simulink model "SimQLPVOFb"  (R2017a)
settings: Solver=VariableStepAuto  StartTime=0.0  StopTime=2000  FixedStep=1e-3  RelTol=1e-3  EnableMultiTasking=on
undefined symbols (not defined in the file): Dr, Du, K, toMpS, toRad, toRPS
libraries: dspsigattribs x3
settings Model: Creator=c00rts11  LastModifiedBy=c00rts11
settings SolverCC: ZeroCrossAlgorithm=Adaptive

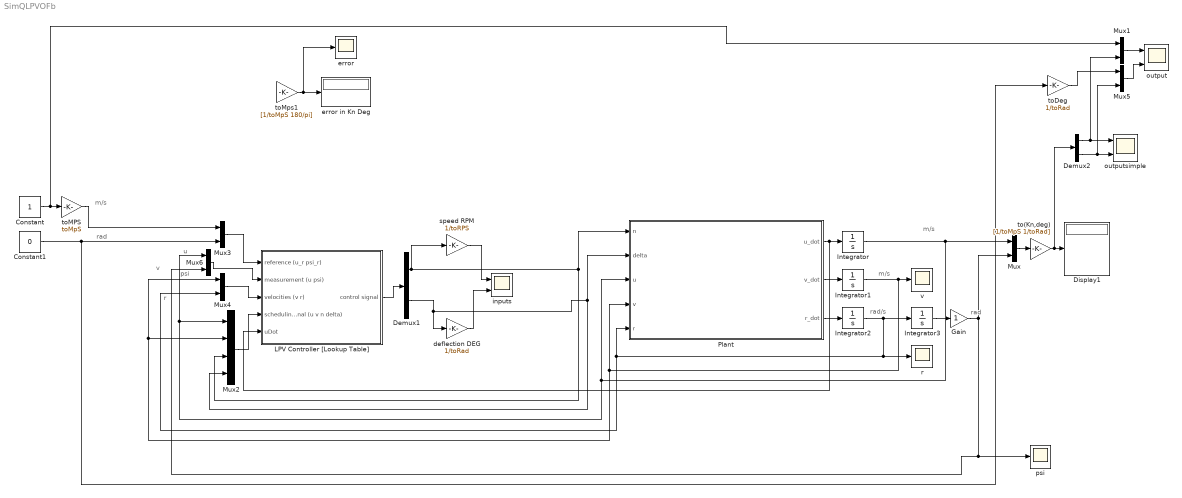
== system SimQLPVOFb ==
  note: psi
  note: u
  note: r
  note: v
  note: rad
  note: rad/s
  note: m/s
  note: m/s
  note: rad
  note: m/s
  Constant : Constant
  Constant1 : Constant  Value=0
  Demux1 : Demux  Outputs=2
  Demux2 : Demux  Outputs=2
  Display1 : Display
  Gain : Gain
  Integrator : Integrator  InitialCondition=.51*toMpS  UpperSaturationLimit=16*toMpS  LowerSaturationLimit=1e-1*toMpS
  Integrator1 : Integrator  LimitOutput=on  UpperSaturationLimit=1*toMpS  LowerSaturationLimit=-1*toMpS
  Integrator2 : Integrator  LimitOutput=on  UpperSaturationLimit=1  LowerSaturationLimit=-1
  Integrator3 : Integrator  InitialCondition=0*toRad  UpperSaturationLimit=180*toRad  LowerSaturationLimit=-180*toRad  WrapState=on  WrappedStateUpperValue=180*toRad  WrappedStateLowerValue=-180*toRad  IgnoreLimit=on
  LPV Controller [Lookup Table] : Subsystem
  Mux{,1,3..6} (6 alike) : Mux  Inputs=2
  Mux2 : Mux
  Plant : MATLAB Function  TreatAsAtomicUnit=on
  deflection DEG : Gain  Gain=1/toRad
  error : Scope
  error in Kn Deg : Display
  inputs : Scope  NumInputPorts=2
  output : Scope  NumInputPorts=2
  outputsimple : Scope  NumInputPorts=2
  psi : Scope
  r : Scope
  speed RPM : Gain  Gain=1/toRPS
  to(Kn,deg) : Gain  Gain=[1/toMpS 1/toRad]
  toDeg : Gain  Gain=1/toRad
  toMPS : Gain  Gain=toMpS
  toMps1 : Gain  Gain=[1/toMpS 180/pi]
  v : Scope
  wires:
  toMPS/1 -> Mux3/1
  Plant/2(v_dot) -> Integrator1/1
  Plant/3(r_dot) -> Integrator2/1
  Plant/1(u_dot) -> LPV Controller [Lookup Table]/5(uDot), Integrator/1
  speed RPM/1 -> inputs/1
  Demux1/1 -> Plant/1(n), Mux2/3, speed RPM/1
  Demux1/2 -> deflection DEG/1, Mux2/4, Plant/2(delta)
  deflection DEG/1 -> inputs/2
  toMps1/1 -> error/1, error in Kn Deg/1
  Integrator/1 -> Mux/1, Mux6/1, Mux2/1, Plant/3(u)
  Integrator2/1 -> Integrator3/1, r/1, Mux4/2, Plant/5(r)
  to(Kn,deg)/1 -> Demux2/1, Display1/1
  Mux/1 -> to(Kn,deg)/1
  Mux5/1 -> output/2
  Mux1/1 -> output/1
  Constant/1 -> Mux1/1, toMPS/1
  toDeg/1 -> Mux5/1
  Demux2/2 -> Mux5/2, outputsimple/2
  Demux2/1 -> Mux1/2, outputsimple/1
  Constant1/1 -> Mux3/2, toDeg/1
  Integrator3/1 -> Gain/1
  Gain/1 -> Mux/2, Mux6/2, psi/1
  Mux2/1 -> LPV Controller [Lookup Table]/4(scheduling signal (u v n delta))
  Mux3/1 -> LPV Controller [Lookup Table]/1(reference (u_r psi_r))
  Mux4/1 -> LPV Controller [Lookup Table]/3(velocities (v r))
  Mux6/1 -> LPV Controller [Lookup Table]/2(measurement (u psi))
  LPV Controller [Lookup Table]/1(control signal) -> Demux1/1
  Integrator1/1 -> Mux2/2, Mux4/1, Plant/4(v), v/1

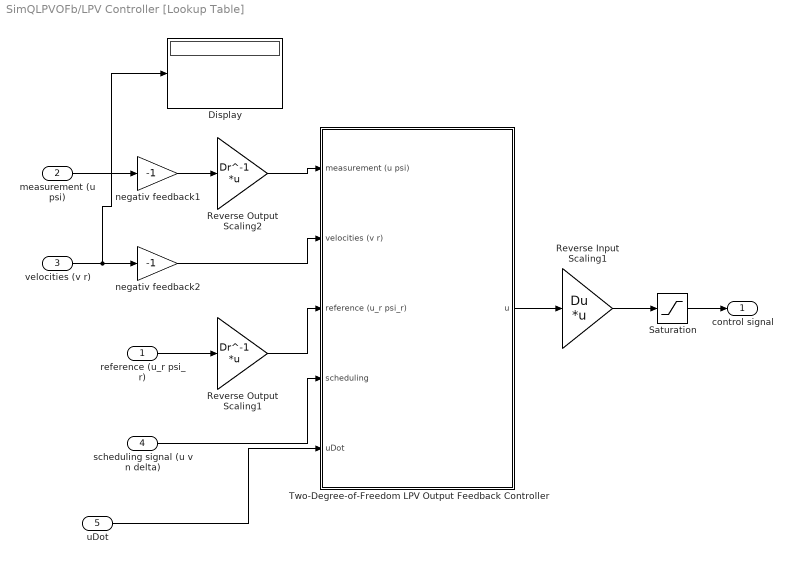
== system SimQLPVOFb/LPV Controller [Lookup Table] ==
  reference (u_r psi_r) : Inport
  measurement (u psi) : Inport  Port=2
  velocities (v r) : Inport  Port=3
  scheduling signal (u v n delta) : Inport  Port=4
  uDot : Inport  Port=5
  Display : Display
  Reverse Input Scaling1 : Gain  Gain=Du  Multiplication=Matrix(K*u)
  Reverse Output Scaling1 : Gain  Gain=Dr^-1  Multiplication=Matrix(K*u)
  Reverse Output Scaling2 : Gain  Gain=Dr^-1  Multiplication=Matrix(K*u)
  Saturation : Saturate  UpperLimit=[20.*toRPS 3.*toRad]  LowerLimit=[-20.*toRPS -3.*toRad]
  Two-Degree-of-Freedom LPV Output Feedback Controller : Subsystem
  negativ feedback1 : Gain  Gain=-1
  negativ feedback2 : Gain  Gain=-1
  control signal : Outport
  wires:
  velocities (v r)/1 -> Display/1, negativ feedback2/1
  scheduling signal (u v n delta)/1 -> Two-Degree-of-Freedom LPV Output Feedback Controller/4(scheduling)
  Reverse Output Scaling2/1 -> Two-Degree-of-Freedom LPV Output Feedback Controller/1(measurement (u psi))
  Two-Degree-of-Freedom LPV Output Feedback Controller/1(u) -> Reverse Input Scaling1/1
  Reverse Input Scaling1/1 -> Saturation/1
  measurement (u psi)/1 -> negativ feedback1/1
  reference (u_r psi_r)/1 -> Reverse Output Scaling1/1
  Reverse Output Scaling1/1 -> Two-Degree-of-Freedom LPV Output Feedback Controller/3(reference (u_r psi_r))
  negativ feedback1/1 -> Reverse Output Scaling2/1
  negativ feedback2/1 -> Two-Degree-of-Freedom LPV Output Feedback Controller/2(velocities (v r))
  Saturation/1 -> control signal/1
  uDot/1 -> Two-Degree-of-Freedom LPV Output Feedback Controller/5(uDot)

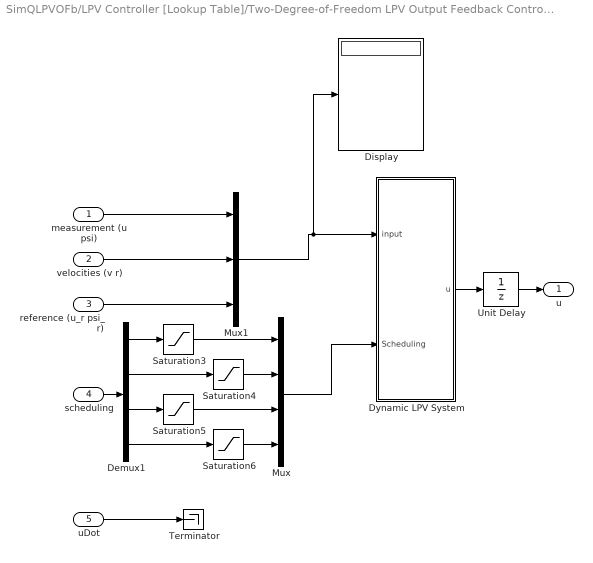
== system SimQLPVOFb/LPV Controller [Lookup Table]/Two-Degree-of-Freedom LPV Output Feedback Controller ==
  measurement (u psi) : Inport
  velocities (v r) : Inport  Port=2
  reference (u_r psi_r) : Inport  Port=3
  scheduling : Inport  Port=4
  uDot : Inport  Port=5
  Demux1 : Demux
  Display : Display
  Dynamic LPV System : Subsystem
  Mux : Mux
  Mux1 : Mux  Inputs=[2 2 2]
  Saturation3 : Saturate  UpperLimit=K.Parameter.u.Range(2)  LowerLimit=K.Parameter.u.Range(1)
  Saturation4 : Saturate  UpperLimit=K.Parameter.v.Range(2)  LowerLimit=K.Parameter.v.Range(1)
  Saturation5 : Saturate  UpperLimit=K.Parameter.n.Range(2)  LowerLimit=K.Parameter.n.Range(1)
  Saturation6 : Saturate  UpperLimit=K.Parameter.delta.Range(2)  LowerLimit=K.Parameter.delta.Range(1)
  Terminator : Terminator
  Unit Delay : UnitDelay  InitialCondition=[1 0]  SampleTime=-1
  u : Outport
  wires:
  velocities (v r)/1 -> Mux1/2
  Dynamic LPV System/1(u) -> Unit Delay/1
  measurement (u psi)/1 -> Mux1/1
  reference (u_r psi_r)/1 -> Mux1/3
  Demux1/4 -> Saturation6/1
  Demux1/3 -> Saturation5/1
  Demux1/1 -> Saturation3/1
  Demux1/2 -> Saturation4/1
  Saturation4/1 -> Mux/2
  Saturation3/1 -> Mux/1
  Saturation5/1 -> Mux/3
  Saturation6/1 -> Mux/4
  Mux/1 -> Dynamic LPV System/2(Scheduling)
  scheduling/1 -> Demux1/1
  Mux1/1 -> Display/1, Dynamic LPV System/1(input)
  Unit Delay/1 -> u/1
  uDot/1 -> Terminator/1

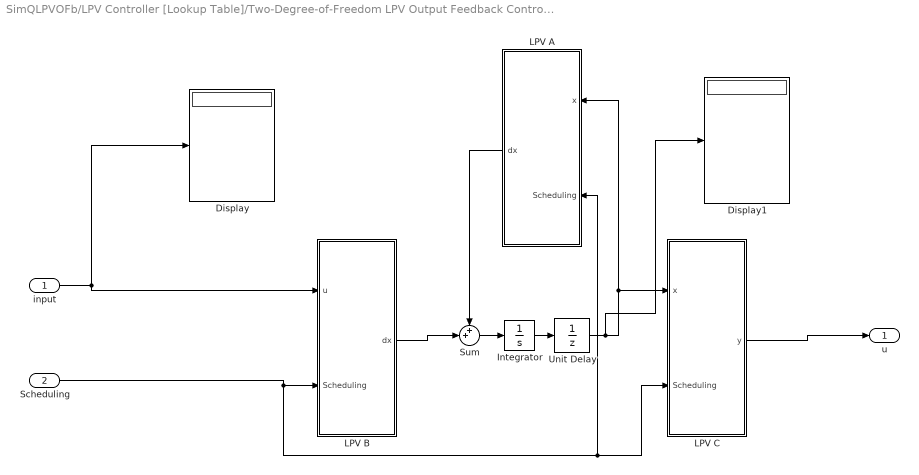
== system SimQLPVOFb/LPV Controller [Lookup Table]/Two-Degree-of-Freedom LPV Output Feedback Controller/Dynamic LPV System ==
  input : Inport
  Scheduling : Inport  Port=2
  Display : Display
  Display1 : Display
  Integrator : Integrator  InitialCondition=zeros(size(K.a,1),1)
  LPV A : Subsystem
  LPV B : Subsystem
  LPV C : Subsystem
  Sum : Sum  Inputs=++|
  Unit Delay : UnitDelay  SampleTime=-1
  u : Outport
  wires:
  LPV C/1(y) -> u/1
  Sum/1 -> Integrator/1
  Integrator/1 -> Unit Delay/1
  input/1 -> Display/1, LPV B/1(u)
  Scheduling/1 -> LPV B/2(Scheduling), LPV A/2(Scheduling), LPV C/2(Scheduling)
  LPV B/1(dx) -> Sum/2
  LPV A/1(dx) -> Sum/1
  Unit Delay/1 -> Display1/1, LPV A/1(x), LPV C/1(x)

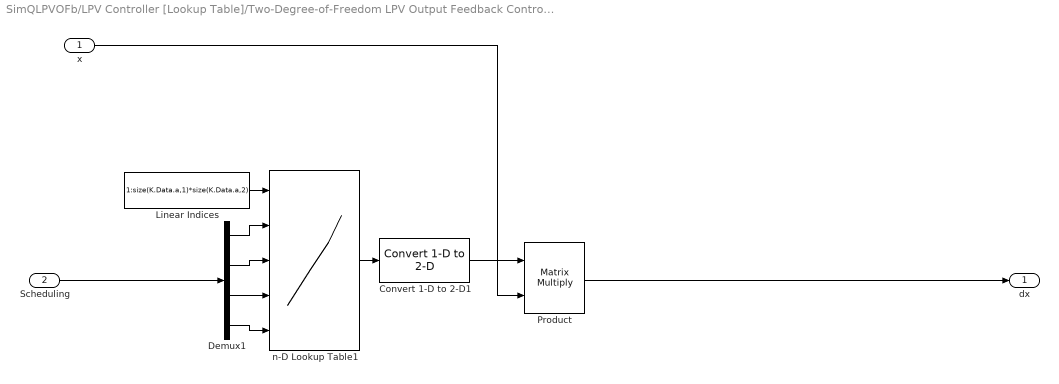
== system SimQLPVOFb/LPV Controller [Lookup Table]/Two-Degree-of-Freedom LPV Output Feedback Controller/Dynamic LPV System/LPV A ==
  x : Inport
  Scheduling : Inport  Port=2
  Convert 1-D to 2-D1 : dspsigattribs/Convert 1-D to 2-D  M=size(K.Data.a,1)  N=size(K.Data.a,2)  frameBasedOut=off
      settings: SourceProductName=DSP System Toolbox  SourceProductBaseCode=DS
  Demux1 : Demux
  Linear Indices : Constant  Value=1:size(K.Data.a,1)*size(K.Data.a,2)
  Product : Product  Multiplication=Matrix(*)
  n-D Lookup Table1 : Lookup_n-D  NumberOfTableDimensions=5  BreakpointsForDimension1=1:size(K.Data.a,1)*size(K.Data.a,2)  BreakpointsForDimension2=K.Parameter.u.GridData  BreakpointsForDimension3=K.Parameter.v.GridData  BreakpointsForDimension4=K.Parameter.n.GridData  BreakpointsForDimension5=K.Parameter.delta.GridData  BreakpointsForDimension6=K.Parameter.uDot.GridData  Table=reshape(K.Data.a,[size(K.Data.a,1)*size(K.Data.a,2), K.Domain.LIVData'])  ExtrapMethod=Clip  UseLastTableValue=on  InternalRulePriority=Speed  RndMeth=Simplest  InputSameDT=on
  dx : Outport
  wires:
  Product/1 -> dx/1
  n-D Lookup Table1/1 -> Convert 1-D to 2-D1/1
  Convert 1-D to 2-D1/1 -> Product/1
  Linear Indices/1 -> n-D Lookup Table1/1
  x/1 -> Product/2
  Scheduling/1 -> Demux1/1
  Demux1/2 -> n-D Lookup Table1/3
  Demux1/1 -> n-D Lookup Table1/2
  Demux1/3 -> n-D Lookup Table1/4
  Demux1/4 -> n-D Lookup Table1/5

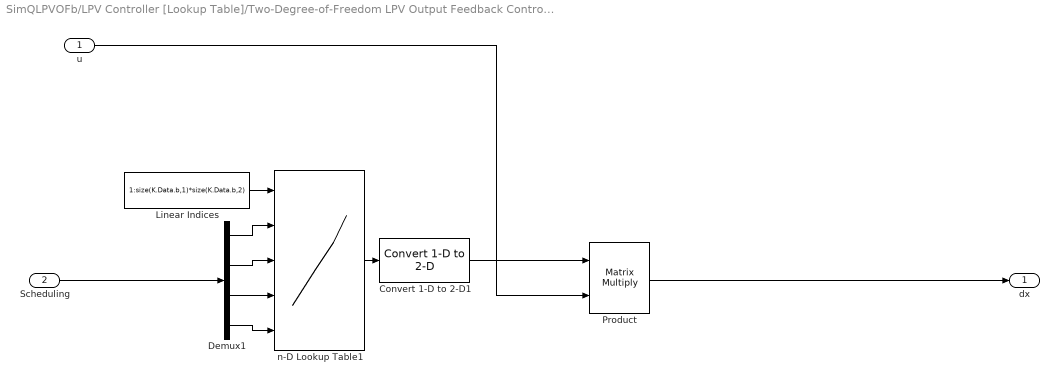
== system SimQLPVOFb/LPV Controller [Lookup Table]/Two-Degree-of-Freedom LPV Output Feedback Controller/Dynamic LPV System/LPV B ==
  u : Inport
  Scheduling : Inport  Port=2
  Convert 1-D to 2-D1 : dspsigattribs/Convert 1-D to 2-D  M=size(K.Data.b,1)  N=size(K.Data.b,2)  frameBasedOut=off
      settings: SourceProductName=DSP System Toolbox  SourceProductBaseCode=DS
  Demux1 : Demux
  Linear Indices : Constant  Value=1:size(K.Data.b,1)*size(K.Data.b,2)
  Product : Product  Multiplication=Matrix(*)
  n-D Lookup Table1 : Lookup_n-D  NumberOfTableDimensions=5  BreakpointsForDimension1=1:size(K.Data.b,1)*size(K.Data.b,2)  BreakpointsForDimension2=K.Parameter.u.GridData  BreakpointsForDimension3=K.Parameter.v.GridData  BreakpointsForDimension4=K.Parameter.n.GridData  BreakpointsForDimension5=K.Parameter.delta.GridData  BreakpointsForDimension6=K.Parameter.uDot.GridData  Table=reshape(K.Data.b,[size(K.Data.b,1)*size(K.Data.b,2), K.Domain.LIVData'])  ExtrapMethod=Clip  UseLastTableValue=on  InternalRulePriority=Speed  RndMeth=Simplest  InputSameDT=on
  dx : Outport
  wires:
  Product/1 -> dx/1
  n-D Lookup Table1/1 -> Convert 1-D to 2-D1/1
  Convert 1-D to 2-D1/1 -> Product/1
  Linear Indices/1 -> n-D Lookup Table1/1
  u/1 -> Product/2
  Scheduling/1 -> Demux1/1
  Demux1/2 -> n-D Lookup Table1/3
  Demux1/1 -> n-D Lookup Table1/2
  Demux1/3 -> n-D Lookup Table1/4
  Demux1/4 -> n-D Lookup Table1/5

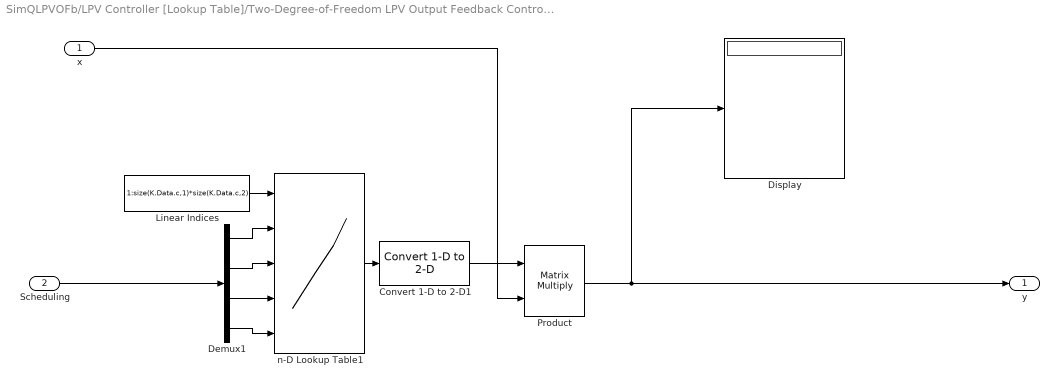
== system SimQLPVOFb/LPV Controller [Lookup Table]/Two-Degree-of-Freedom LPV Output Feedback Controller/Dynamic LPV System/LPV C ==
  x : Inport
  Scheduling : Inport  Port=2
  Convert 1-D to 2-D1 : dspsigattribs/Convert 1-D to 2-D  M=size(K.Data.c,1)  N=size(K.Data.c,2)  frameBasedOut=off
      settings: SourceProductName=DSP System Toolbox  SourceProductBaseCode=DS
  Demux1 : Demux
  Display : Display
  Linear Indices : Constant  Value=1:size(K.Data.c,1)*size(K.Data.c,2)
  Product : Product  Multiplication=Matrix(*)
  n-D Lookup Table1 : Lookup_n-D  NumberOfTableDimensions=5  BreakpointsForDimension1=1:size(K.Data.c,1)*size(K.Data.c,2)  BreakpointsForDimension2=K.Parameter.u.GridData  BreakpointsForDimension3=K.Parameter.v.GridData  BreakpointsForDimension4=K.Parameter.n.GridData  BreakpointsForDimension5=K.Parameter.delta.GridData  BreakpointsForDimension6=K.Parameter.uDot.GridData  Table=reshape(K.Data.c,[size(K.Data.c,1)*size(K.Data.c,2), K.Domain.LIVData'])  ExtrapMethod=Clip  UseLastTableValue=on  InternalRulePriority=Speed  RndMeth=Simplest  InputSameDT=on
  y : Outport
  wires:
  Demux1/1 -> n-D Lookup Table1/2
  Demux1/2 -> n-D Lookup Table1/3
  Demux1/3 -> n-D Lookup Table1/4
  Scheduling/1 -> Demux1/1
  x/1 -> Product/2
  Linear Indices/1 -> n-D Lookup Table1/1
  Convert 1-D to 2-D1/1 -> Product/1
  n-D Lookup Table1/1 -> Convert 1-D to 2-D1/1
  Demux1/4 -> n-D Lookup Table1/5
  Product/1 -> y/1, Display/1

== matlab function SimQLPVOFb/Plant ==
  data: n input; delta input; u input; u_dot output; v input; r input; v_dot output; r_dot output
function [u_dot,v_dot,r_dot] = fcn(n,delta,u,v,r)
% n = n/60;
% v = 0;
% r = 0;
if (u==0)
    u = 1e-1;
end
% Normalization variables
L   =  304.8;          % length of ship (m)
g   =  9.8;            % acceleration of gravity (m/s^2)

% Parameters, hydrodynamic derivatives and main dimensions
% delta_max  = 10;       % max rudder angle      (deg)
% Ddelta_max = 2.33;     % max rudder derivative (deg/s)
% n_max      = 80;       % max shaft velocity    (rpm)

t   =  0.22;
Tm  =  50;
T   =  18.46;

cun =  0.605;  
cnn =  38.2;

Tuu = -0.00695;
Tun = -0.00063;
Tnn =  0.0000354;

m11 =  1.050;          % 1 - Xudot
m22 =  2.020;          % 1 - Yvdot
m33 =  0.1232;         % kz^2 - Nrdot

d11 =  2.020;          % 1 + Xvr
d22 = -0.752;          % Yur - 1
d33 = -0.231;          % Nur - xG 

Xuuz   = -0.0061;   YT     =  0.04;   NT      = -0.02;
Xuu    = -0.0377;   Yvv    = -2.400;  Nvr     = -0.300;
Xvv    =  0.3;      Yuv    = -1.205;  Nuv     = -0.451;   
Xudotz = -0.05;     Yvdotz = -0.387;  Nrdotz  = -0.0045;
Xuuz   = -0.0061;   Yurz   =  0.182;  Nurz    = -0.047;
Xvrz   =  0.387;    Yvvz   = -1.5;    Nvrz    = -0.120;
Xccdd  = -0.093;    Yuvz   =  0;      Nuvz    = -0.241;
Xccbd  =  0.152;    Yccd   =  0.208;  Nccd    = -0.098;
Xvvzz  =  0.0125;   Yccbbd = -2.16;   Nccbbd  =  0.688;
                    Yccbbdz= -0.191;  Nccbbdz =  0.344;

z = T./(50 - T);

% Forces and moments
beta = v/u;
gT   = (1/L*Tuu*u^2 + Tun*u*n + L*Tnn*abs(n)*n);
% C = (cun*u*n + cnn*n^2)*sign(cun*u*n + cnn*n^2);
C = (cun*u*n + cnn*n^2);

gX   = 1/L*(Xuu*u^2 + L*d11*v*r + Xvv*v^2 + Xccdd*C*delta^2 ...
     + Xccbd*C*beta*delta + L*gT*(1-t) + Xuuz*u^2*z ...
     + L*Xvrz*v*r*z + Xvvzz*v^2*z^2);

gY   = 1/L*(Yuv*u*v + Yvv*abs(v)*v + Yccd*C*delta + L*d22*u*r ...
     + Yccbbd*C*abs(beta)*beta*abs(delta) + YT*gT*L ...
     + L*Yurz*u*r*z + Yuvz*u*v*z + Yvvz*abs(v)*v*z  ...
     + Yccbbdz*C*abs(beta)*beta*abs(delta)*z);     

gLN  = Nuv*u*v + L*Nvr*abs(v)*r + Nccd*C*delta +L*d33*u*r ...
     + Nccbbd*C*abs(beta)*beta*abs(delta) + L*NT*gT ...
     + L*Nurz*u*r*z + Nuvz*u*v*z + L*Nvrz*abs(v)*r*z ...
     + Nccbbdz*C*abs(beta)*beta*abs(delta)*z;
 
%  c    = sqrt(cun*u*n + cnn*n^2);
% 
% gX   = 1/L*(Xuu*u^2 + L*d11*v*r + Xvv*v^2 + Xccdd*abs(c)*c*delta^2 ...
%      + Xccbd*abs(c)*c*beta*delta + L*gT*(1-t) + Xuuz*u^2*z ...
%      + L*Xvrz*v*r*z + Xvvzz*v^2*z^2);
% 
% gY   = 1/L*(Yuv*u*v + Yvv*abs(v)*v + Yccd*abs(c)*c*delta + L*d22*u*r ...
%      + Yccbbd*abs(c)*c*abs(beta)*beta*abs(delta) + YT*gT*L ...
%      + L*Yurz*u*r*z + Yuvz*u*v*z + Yvvz*abs(v)*v*z  ...
%      + Yccbbdz*abs(c)*c*abs(beta)*beta*abs(delta)*z);     
% 
% gLN  = Nuv*u*v + L*Nvr*abs(v)*r + Nccd*abs(c)*c*delta +L*d33*u*r ...
%      + Nccbbd*abs(c)*c*abs(beta)*beta*abs(delta) + L*NT*gT ...
%      + L*Nurz*u*r*z + Nuvz*u*v*z + L*Nvrz*abs(v)*r*z ...
%      + Nccbbdz*abs(c)*c*abs(beta)*beta*abs(delta)*z;

m11 = (m11 - Xudotz*z);
m22 = (m22 - Yvdotz*z);
m33 = (m33 - Nrdotz*z);

% Dimensional state derivative
u_dot = gX/m11;
v_dot = gY/m22;
r_dot = gLN/(L^2*m33);
